simulink model "ale"  (R2022a)
settings: Solver=FixedStepAuto  StartTime=0.0  StopTime=10.0  FixedStep=framePeriod_s  RelTol=1e-3
undefined symbols (not defined in the file or in its folder): Aircraft, fire, framePeriod_s, led, throttle, turn
libraries: simulink x14, slpidlib x4, dspfdesign x1
(part 1 of 2)
settings Model: Creator=brian  LastModifiedBy=tuan
settings SolverCC: AlgebraicLoopSolver=TrustRegion
settings OptimizationCC: DefaultParameterBehavior=Inlined  GainParamInheritBuiltInType=on  UseFloatMulNetSlope=on  DefaultUnderspecifiedDataType=single  InlineInvariantSignals=on  PassReuseOutputArgsAs=Individual arguments  ZeroExternalMemoryAtStartup=off  ZeroInternalMemoryAtStartup=off  NoFixptDivByZeroProtection=on  EfficientFloat2IntCast=on  LifeSpan=1  OptimizeBlockOrder=speed  DifferentSizesBufferReuse=on  EfficientTunableParamExpr=on
settings DebuggingCC: ParameterTunabilityLossMsg=error  UnconnectedInputMsg=warning  UnconnectedOutputMsg=warning  UnconnectedLineMsg=warning  SFMachineParentedDataDiag=warning
settings HardwareCC: ProdBitPerPointer=32  ProdBitPerSizeT=32  ProdBitPerPtrDiffT=32  ProdLargestAtomicInteger=Long  ProdLargestAtomicFloat=Double  ProdWordSize=32  ProdLongLongMode=on  ProdHWDeviceType=NXP->Cortex-M4
settings ModelReferenceCC: ModelReferenceNumInstancesAllowed=Single
settings SFSimCC: SimParseCustomCode=off  MATLABDynamicMemAlloc=off
settings RTWCC: SystemTargetFile=ert.tlc  GenCodeOnly=on  TemplateMakefile=ert_default_tmf  RTWVerbose=off  BuildConfiguration=Faster Runs  TargetLang=C++  DLArmComputeVersion=19.05
settings CodeAppCC: ForceParamTrailComments=on  IgnoreCustomStorageClasses=off  OperatorAnnotations=on  SimulinkDataObjDesc=on  SFDataObjDesc=on  CustomSymbolStrGlobalVar=rt$N$M  CustomSymbolStrType=$N$M  CustomSymbolStrFcn=$N$M$F  CustomSymbolStrMacro=$N$M  InsertBlockDesc=on
settings ERTTargetCC: TargetLangStandard=C++03 (ISO)  IncludeMdlTerminateFcn=off  CombineSignalStateStructs=on  SuppressErrorStatus=on  SupportAbsoluteTime=off  CodeInterfacePackaging=C++ class  SupportNonFinite=off  SupportComplex=off  ERTHeaderFileRootName=autocode$E  ERTSourceFileRootName=autocode$E  InlinedParameterPlacement=NonHierarchical  RootIOFormat=Structure reference  ERTCustomFileTemplate=example_file_process.tlc  ERTFilePackagingFormat=Compact  ArrayContainerType=std::array

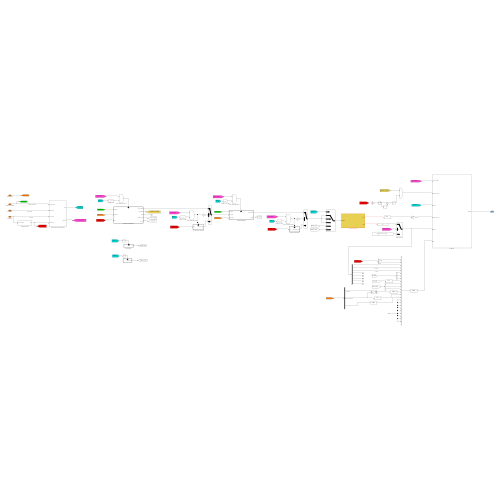
[thumbnail: Simulink's stored preview of the top-level diagram]
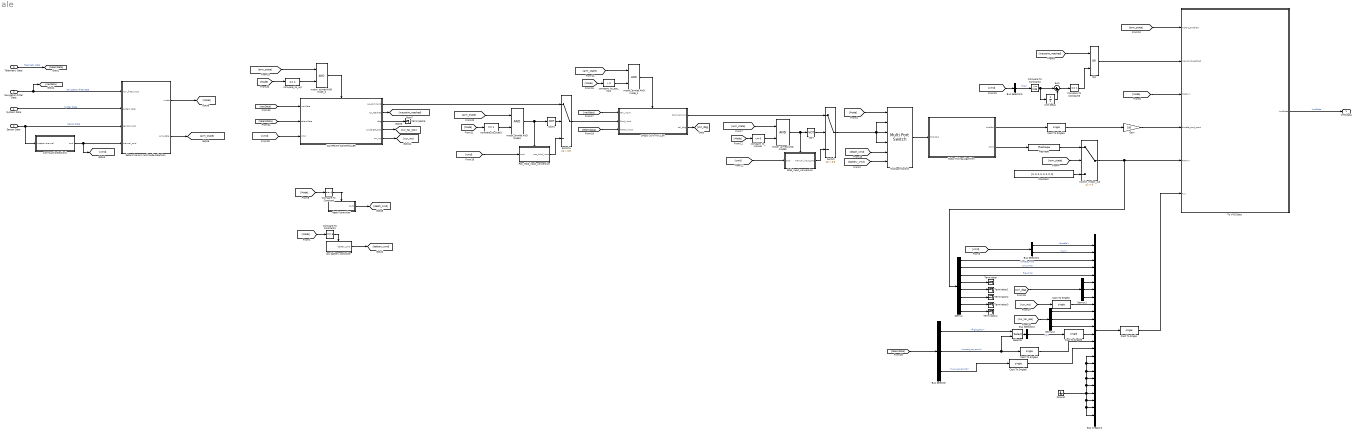
== system ale ==
  System Data : Inport  OutDataTypeStr=Bus: SysData  SampleTime=framePeriod_s  BusOutputAsStruct=on
  Sensor Data : Inport  Port=2  OutDataTypeStr=Bus: SensorData  SampleTime=framePeriod_s  BusOutputAsStruct=on
  Navigation Filter Data : Inport  Port=3  OutDataTypeStr=Bus: NavData  SampleTime=framePeriod_s  BusOutputAsStruct=on
  Telemetry Data : Inport  Port=4  OutDataTypeStr=Bus: TelemData  SampleTime=framePeriod_s  BusOutputAsStruct=on
  Bus Creator2 : BusCreator  Inputs=24
  Bus Selector : BusSelector  OutputSignals=flight_plan,current_waypoint,num_waypoints
  Bus Selector1 : BusSelector  OutputSignals=throttle,turn
  Bus Selector2 : BusSelector  OutputSignals=x
  Bus Selector3 : BusSelector  OutputSignals=fire
  Cast To Single{,1..5} (6 alike) : DataTypeConversion  OutDataTypeStr=single  SaturateOnIntegerOverflow=off  RndMeth=Floor
  Compare To Constant : simulink/Logic and Bit Operations/Compare To Constant  relop===  const=4  OutDataTypeStr=boolean
  Compare To Constant1 : simulink/Logic and Bit Operations/Compare To Constant  relop===  const=3  OutDataTypeStr=boolean
  Compare To Constant2 : simulink/Logic and Bit Operations/Compare To Constant  relop=>=  const=0.99  OutDataTypeStr=uint8
  Compare To Constant3 : simulink/Logic and Bit Operations/Compare To Constant  relop===  const=1  OutDataTypeStr=boolean
  Constant : Constant  Value=[0, 0, 0, 0, 0, 0, 0, 0]  OutDataTypeStr=single  SampleTime=framePeriod_s
  Demux : Demux  Outputs=8
  Demux1 : Demux  Outputs=3
  Demux2 : Demux  Outputs=3
  Gain : Gain  Gain=100
  Ground : Ground
  Motor Mixing Algorithm : Subsystem
  Multiport Switch : MultiPortSwitch  DataPortOrder=Specify indices  DataPortIndices={0, 1, 2, 3, 4}  DiagnosticForDefault=None  SaturateOnIntegerOverflow=off  InputSameDT=off
  NOT : Logic  Operator=NOT  IconShape=distinctive  AllPortsSameDT=off  OutDataTypeStr=boolean
  NOT1 : Logic  Operator=NOT  IconShape=distinctive  AllPortsSameDT=off  OutDataTypeStr=boolean
  OR : Logic  Operator=OR  IconShape=distinctive  AllPortsSameDT=off  OutDataTypeStr=boolean
  Pos_Hold_input_conversion : Subsystem
  Reshape : Reshape
  SPEED CONTROLLER : Subsystem
  Selector : Selector  IndexMode=Zero-based  InputPortWidth=100  IndexOptions=Index vector (port)  Indices=[1 3]  OutputSizes=1
  Stab_input_conversion : Subsystem
  Sum : Sum  Inputs=|+-
  Switch : Switch  Criteria=u2 > Threshold  Threshold=0.5  SaturateOnIntegerOverflow=off  InputSameDT=off
  Switch1 : Switch  Criteria=u2 > Threshold  Threshold=0.5  SaturateOnIntegerOverflow=off  InputSameDT=off
  Terminator{,1..5} (6 alike) : Terminator
  To VMS Data : Subsystem
  Unit Delay : UnitDelay  SampleTime=-1  HasFrameUpgradeWarning=on
  WAYPOINT CONTROLLER : Subsystem
  command selection1 : Subsystem
  compare_to_manual : simulink/Logic and Bit Operations/Compare To Constant  relop=<=  const=0  OutDataTypeStr=boolean
  compare_to_pos_hold : simulink/Logic and Bit Operations/Compare To Constant  relop=>  const=0  OutDataTypeStr=boolean
  compare_to_stab1 : simulink/Logic and Bit Operations/Compare To Constant  relop===  const=1  OutDataTypeStr=boolean
  compare_to_wp : simulink/Logic and Bit Operations/Compare To Constant  relop===  const=2  OutDataTypeStr=boolean
  death controller : Subsystem
  determine arm and mode selection : Subsystem
  low battery controller : Subsystem  TreatAsAtomicUnit=on
  motor_armed AND mode0 : Logic  IconShape=distinctive  AllPortsSameDT=off  OutDataTypeStr=boolean
  motor_armed AND mode1 : Logic  IconShape=distinctive  AllPortsSameDT=off  OutDataTypeStr=boolean
  motor_armed AND mode_1 : Logic  IconShape=distinctive  AllPortsSameDT=off  OutDataTypeStr=boolean
  motor_armed AND mode_2 : Logic  IconShape=distinctive  AllPortsSameDT=off  OutDataTypeStr=boolean
  switch_motor_out : Switch  Criteria=u2 > Threshold  SaturateOnIntegerOverflow=off  InputSameDT=off
  VMS Data : Outport  OutDataTypeStr=Bus: VmsData  SampleTime=framePeriod_s  BusOutputAsStruct=on
  wires:
  [Mode] -> To VMS Data/3(Mode in)
  Gain/1 -> To VMS Data/4(throttle_cmd_prcnt)
  Reshape/1 -> switch_motor_out/1
  Bus Selector1/1 -> Bus Creator2/1  "<throttle>"
  [arm_state] -> To VMS Data/1(motors_enabled)
  Ground/1 -> Bus Creator2/16, Bus Creator2/17, Bus Creator2/18, Bus Creator2/19, Bus Creator2/20, Bus Creator2/21, Bus Creator2/24, Bus Creator2/23, Bus Creator2/22
  [arm_state] -> switch_motor_out/2
  switch_motor_out/1 -> Demux/1, To VMS Data/5(PWM In)
  Constant/1 -> switch_motor_out/3
  Cast To Single/1 -> To VMS Data/6(Aux)
  Bus Creator2/1 -> Cast To Single/1
  Motor Mixing Algorithm/1(throttle) -> Cast To Single1/1
  Motor Mixing Algorithm/2(PWM) -> Reshape/1
  Cast To Single1/1 -> Gain/1
  To VMS Data/1(VmsData) -> VMS Data/1  "VmsData"
  Sensor Data/1 -> determine arm and mode selection/3(sensor_input), command selection1/1(inceptor channel)  "Sensor Data"
  Telemetry Data/1 -> [telemData]  "Telemetry Data"
  determine arm and mode selection/1(mode) -> [Mode]
  System Data/1 -> determine arm and mode selection/2(system data)  "Systen Data"
  determine arm and mode selection/2(arm_state) -> [arm_state]
  Navigation Filter Data/1 -> [navData], determine arm and mode selection/1(nav_filter_input)  "Navigation Filter Data"
  [cmd] -> Bus Selector1/1
  Bus Selector1/2 -> Bus Creator2/2  "<turn>"
  Demux/1 -> Bus Creator2/3  "throttle_mma"
  Demux/2 -> Bus Creator2/4  "turn_mma"
  Demux/3 -> Bus Creator2/5  "fire_mma"
  Demux/4 -> Terminator/1
  Demux/5 -> Terminator1/1
  Demux/6 -> Terminator2/1
  Demux/7 -> Terminator3/1
  Demux/8 -> Terminator4/1
  [Mode] -> Multiport Switch/1
  death controller/1(Out1) -> [death_cmd]
  [Mode] -> Compare To Constant/1
  Compare To Constant/1 -> death controller/Enable
  [Mode] -> Compare To Constant1/1
  Compare To Constant1/1 -> low battery controller/Enable
  low battery controller/1(battery_cmd) -> [battery_cmd]
  command selection1/1(cmd) -> determine arm and mode selection/4(manual_cmd), [cmd]
  Switch/1 -> Multiport Switch/2, Multiport Switch/4, Multiport Switch/3
  [Mode] -> compare_to_manual/1
  compare_to_manual/1 -> motor_armed AND mode0/2
  motor_armed AND mode0/1 -> Stab_input_conversion/Enable, NOT/1
  [arm_state] -> motor_armed AND mode0/1
  NOT/1 -> Switch/2
  [cmd] -> Stab_input_conversion/1(cmd)
  Stab_input_conversion/1(manual_input_cmd) -> Switch/3
  [navData] -> SPEED CONTROLLER/1(Nav_input)
  compare_to_pos_hold/1 -> motor_armed AND mode_1/2
  [arm_state] -> motor_armed AND mode_1/1
  [Mode] -> compare_to_pos_hold/1
  motor_armed AND mode_1/1 -> SPEED CONTROLLER/Enable
  SPEED CONTROLLER/1(Command out) -> Switch/1
  [Mode] -> compare_to_stab1/1
  motor_armed AND mode1/1 -> Pos_Hold_input_conversion/Enable, NOT1/1
  Switch1/1 -> SPEED CONTROLLER/2(Cmd_input)
  Pos_Hold_input_conversion/1(pos_hold_input) -> Switch1/3
  compare_to_stab1/1 -> motor_armed AND mode1/2
  NOT1/1 -> Switch1/2
  [cmd] -> Pos_Hold_input_conversion/1(cmd)
  [arm_state] -> motor_armed AND mode1/1
  [telemData] -> SPEED CONTROLLER/3(Telem_input)
  Multiport Switch/1 -> Motor Mixing Algorithm/1(MMA Bus)
  WAYPOINT CONTROLLER/1(wp_command) -> Switch1/1
  WAYPOINT CONTROLLER/2(wp_reached) -> [waypoint_reached]
  WAYPOINT CONTROLLER/3(dbg) -> Terminator5/1
  [arm_state] -> motor_armed AND mode_2/1
  compare_to_wp/1 -> motor_armed AND mode_2/2
  [Mode] -> compare_to_wp/1
  motor_armed AND mode_2/1 -> WAYPOINT CONTROLLER/Enable
  [telemData] -> WAYPOINT CONTROLLER/2(telemData)
  [navData] -> WAYPOINT CONTROLLER/1(navData)
  [cmd] -> WAYPOINT CONTROLLER/3(cmd)
  [battery_cmd] -> Multiport Switch/6
  [death_cmd] -> Multiport Switch/5
  SPEED CONTROLLER/2(ctrl_dbg) -> [ctrl_dbg]
  [ctrl_dbg] -> Demux1/1
  Demux1/1 -> Bus Creator2/6
  Demux1/2 -> Bus Creator2/7
  Demux1/3 -> Bus Creator2/8
  WAYPOINT CONTROLLER/4(cur_target_pos) -> [cur_tar_pos]
  WAYPOINT CONTROLLER/5(cur_wp) -> [cur_wp]
  [cur_wp] -> Cast To Single2/1
  Demux2/3 -> Bus Creator2/12
  Demux2/2 -> Bus Creator2/11
  Demux2/1 -> Bus Creator2/10
  [cur_tar_pos] -> Demux2/1
  Cast To Single2/1 -> Bus Creator2/9
  [telemData] -> Bus Selector/1
  Bus Selector/1 -> Selector/1  "<flight_plan>"
  Selector/1 -> Bus Selector2/1
  Bus Selector2/1 -> Cast To Single3/1  "<x>"
  Cast To Single3/1 -> Bus Creator2/13
  Bus Selector/2 -> Selector/2, Cast To Single4/1  "<current_waypoint>"
  [waypoint_reached] -> OR/1
  OR/1 -> To VMS Data/2(waypoint_reached)
  [cmd] -> Bus Selector3/1
  Bus Selector3/1 -> Compare To Constant2/1  "<fire>"
  Bus Selector/3 -> Cast To Single5/1  "<num_waypoints>"
  Cast To Single4/1 -> Bus Creator2/14
  Cast To Single5/1 -> Bus Creator2/15
  Compare To Constant2/1 -> Sum/1, Unit Delay/1
  Compare To Constant3/1 -> OR/2
  Sum/1 -> Compare To Constant3/1
  Unit Delay/1 -> Sum/2

== system ale/Motor Mixing Algorithm ==
  note: Other outputs are for fun things like Laser, Death or alive signal and speeker
  note: Motor output command is from -1 to 1
  note: this block map the control input to the correct hardware output signal. ie speed and turn command to the corresponding wheel speeds
  MMA Bus : Inport
  Bus Selector : BusSelector  OutputSignals=throttle,turn,fire,led
  Motor Mix : Constant  Value=Aircraft.Motor.mix  OutDataTypeStr=single  SampleTime=framePeriod_s
  Multiply : Product  Inputs=**  Multiplication=Matrix(*)  OutDataTypeStr=single
  Mux : Mux
  Reshape : Reshape  OutputDimensionality=Column vector (2-D)
  Saturation : Saturate  UpperLimit=1  LowerLimit=-1
  throttle : Outport
  PWM : Outport  Port=2
  wires:
  Mux/1 -> Reshape/1
  MMA Bus/1 -> Bus Selector/1
  Bus Selector/1 -> throttle/1, Mux/1  "<throttle>"
  Bus Selector/2 -> Mux/2  "<turn>"
  Multiply/1 -> Saturation/1  "Command"
  Reshape/1 -> Multiply/2
  Motor Mix/1 -> Multiply/1
  Bus Selector/3 -> Mux/3  "<fire>"
  Saturation/1 -> PWM/1
  Bus Selector/4 -> Mux/4  "<led>"

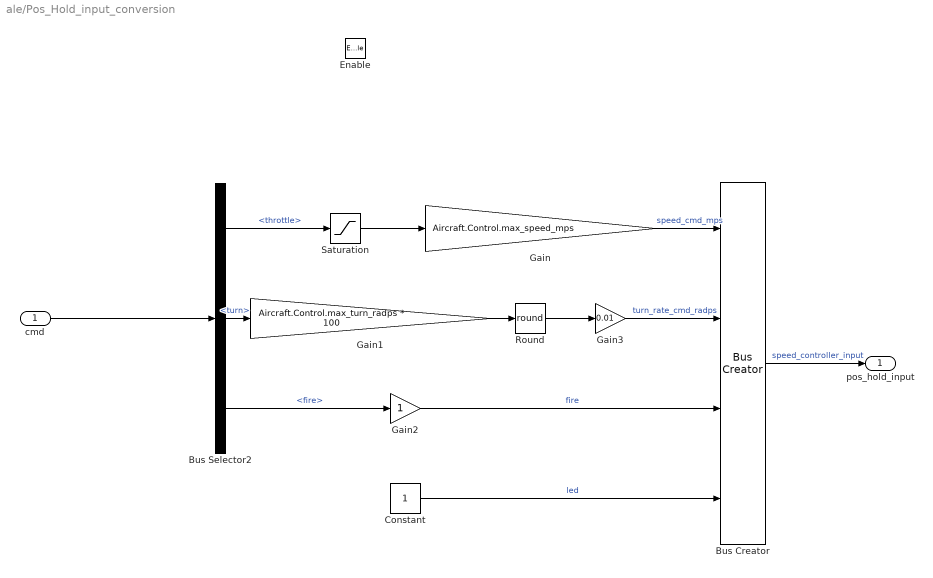
== system ale/Pos_Hold_input_conversion ==
  cmd : Inport
  Enable : EnablePort
  Bus Creator : BusCreator  Inputs=4
  Bus Selector2 : BusSelector  OutputSignals=throttle,turn,fire
  Constant : Constant  OutDataTypeStr=single
  Gain : Gain  Gain=Aircraft.Control.max_speed_mps
  Gain1 : Gain  Gain=Aircraft.Control.max_turn_radps * 100
  Gain2 : Gain
  Gain3 : Gain  Gain=0.01
  Round : Rounding  Operator=round
  Saturation : Saturate  UpperLimit=1  LowerLimit=0
  pos_hold_input : Outport
  wires:
  Bus Selector2/2 -> Gain1/1  "<turn>"
  Bus Creator/1 -> pos_hold_input/1  "speed_controller_input"
  Gain2/1 -> Bus Creator/3  "fire"
  Gain/1 -> Bus Creator/1  "speed_cmd_mps"
  Bus Selector2/3 -> Gain2/1  "<fire>"
  Constant/1 -> Bus Creator/4  "led"
  Bus Selector2/1 -> Saturation/1  "<throttle>"
  cmd/1 -> Bus Selector2/1
  Gain1/1 -> Round/1
  Round/1 -> Gain3/1
  Gain3/1 -> Bus Creator/2  "turn_rate_cmd_radps"
  Saturation/1 -> Gain/1

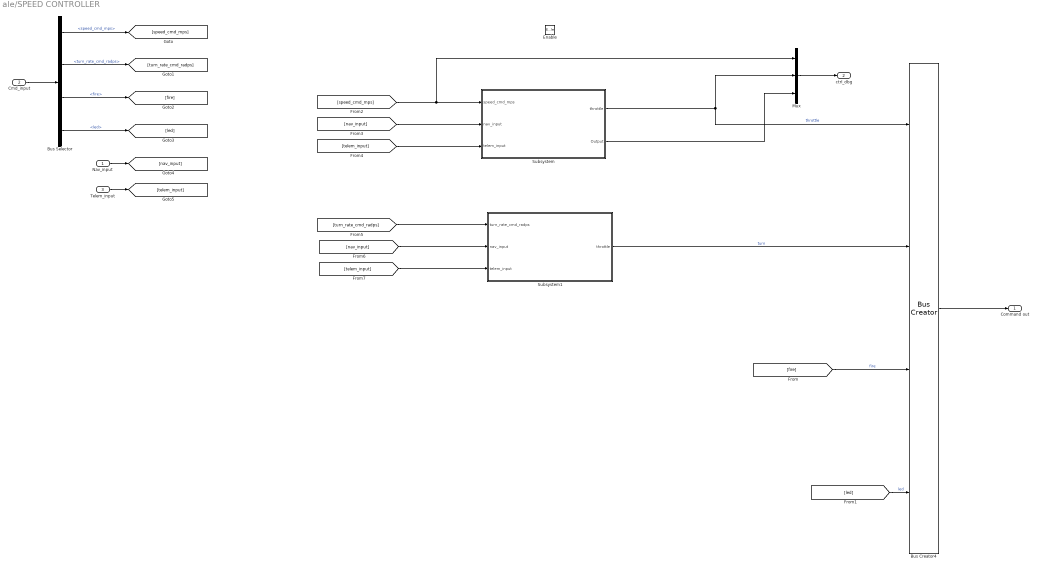
== system ale/SPEED CONTROLLER ==
  Nav_input : Inport
  Cmd_input : Inport  Port=2
  Telem_input : Inport  Port=3
  Enable : EnablePort  PropagateVarSize=During execution
  Bus Creator4 : BusCreator  Inputs=throttle,turn,fire,led
  Bus Selector : BusSelector  OutputSignals=speed_cmd_mps,turn_rate_cmd_radps,fire,led
  Mux : Mux  Inputs=3
  Subsystem : Subsystem
  Subsystem1 : Subsystem
  Command out : Outport
  ctrl_dbg : Outport  Port=2
  wires:
  Bus Creator4/1 -> Command out/1
  Cmd_input/1 -> Bus Selector/1
  [led] -> Bus Creator4/4  "led"
  Subsystem1/1(throttle) -> Bus Creator4/2  "turn"
  [fire] -> Bus Creator4/3  "fire"
  Bus Selector/1 -> [speed_cmd_mps]  "<speed_cmd_mps>"
  Bus Selector/4 -> [led]  "<led>"
  Bus Selector/3 -> [fire]  "<fire>"
  Bus Selector/2 -> [turn_rate_cmd_radps]  "<turn_rate_cmd_radps>"
  [speed_cmd_mps] -> Mux/1, Subsystem/1(speed_cmd_mps)
  Subsystem/1(throttle) -> Bus Creator4/1, Mux/2  "throttle"
  Nav_input/1 -> [nav_input]
  Telem_input/1 -> [telem_input]
  [nav_input] -> Subsystem/2(nav_input)
  [telem_input] -> Subsystem/3(telem_input)
  [turn_rate_cmd_radps] -> Subsystem1/1(turn_rate_cmd_radps)
  [nav_input] -> Subsystem1/2(nav_input)
  [telem_input] -> Subsystem1/3(telem_input)
  Mux/1 -> ctrl_dbg/1
  Subsystem/2(Output) -> Mux/3

== system ale/Stab_input_conversion ==
  cmd : Inport
  Enable : EnablePort
  Bus Creator : BusCreator  Inputs=4
  Bus Selector2 : BusSelector  OutputSignals=throttle,turn,fire
  Constant : Constant  OutDataTypeStr=single  SampleTime=framePeriod_s
  Gain : Gain
  Gain1 : Gain
  Gain2 : Gain
  manual_input_cmd : Outport
  wires:
  Bus Selector2/2 -> Gain1/1  "<turn>"
  Bus Creator/1 -> manual_input_cmd/1  "manual_input"
  Gain1/1 -> Bus Creator/2  "turn"
  cmd/1 -> Bus Selector2/1
  Bus Selector2/1 -> Gain/1  "<throttle>"
  Gain/1 -> Bus Creator/1  "throttle"
  Gain2/1 -> Bus Creator/3  "fire"
  Bus Selector2/3 -> Gain2/1  "<fire>"
  Constant/1 -> Bus Creator/4  "led"

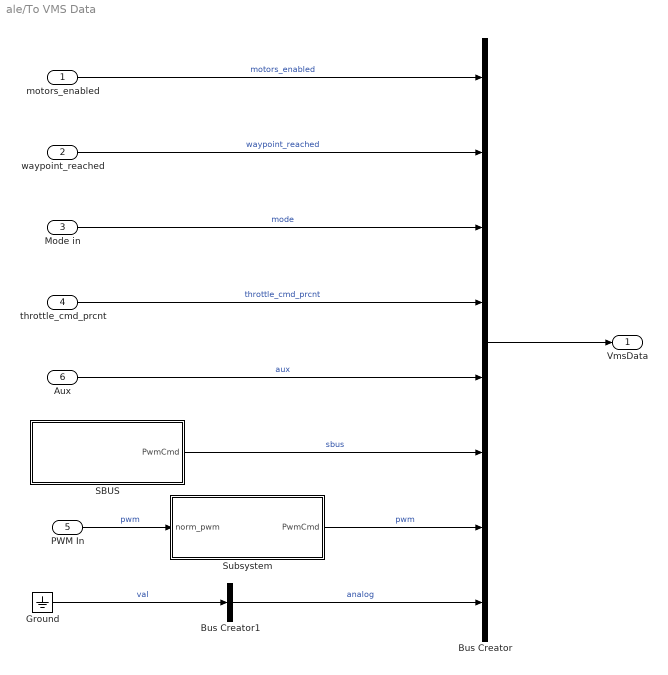
== system ale/To VMS Data ==
  motors_enabled : Inport
  waypoint_reached : Inport  Port=2
  Mode in : Inport  Port=3
  throttle_cmd_prcnt : Inport  Port=4
  PWM In : Inport  Port=5
  Aux : Inport  Port=6
  Bus Creator : BusCreator  Inputs=8  OutDataTypeStr=Bus: VmsData  NonVirtualBus=on
  Bus Creator1 : BusCreator  Inputs=1  OutDataTypeStr=Bus: AnalogData
  Ground : Ground
  "SBUS " : Subsystem
  Subsystem : Subsystem
  VmsData : Outport
  wires:
  waypoint_reached/1 -> Bus Creator/2  "waypoint_reached"
  Mode in/1 -> Bus Creator/3  "mode"
  motors_enabled/1 -> Bus Creator/1  "motors_enabled"
  Bus Creator/1 -> VmsData/1
  throttle_cmd_prcnt/1 -> Bus Creator/4  "throttle_cmd_prcnt"
  PWM In/1 -> Subsystem/1(norm_pwm)  "pwm"
  Subsystem/1(PwmCmd) -> Bus Creator/7  "pwm"
  Bus Creator1/1 -> Bus Creator/8  "analog"
  Ground/1 -> Bus Creator1/1  "val"
  Aux/1 -> Bus Creator/5  "aux"
  "SBUS "/1(PwmCmd) -> Bus Creator/6  "sbus"

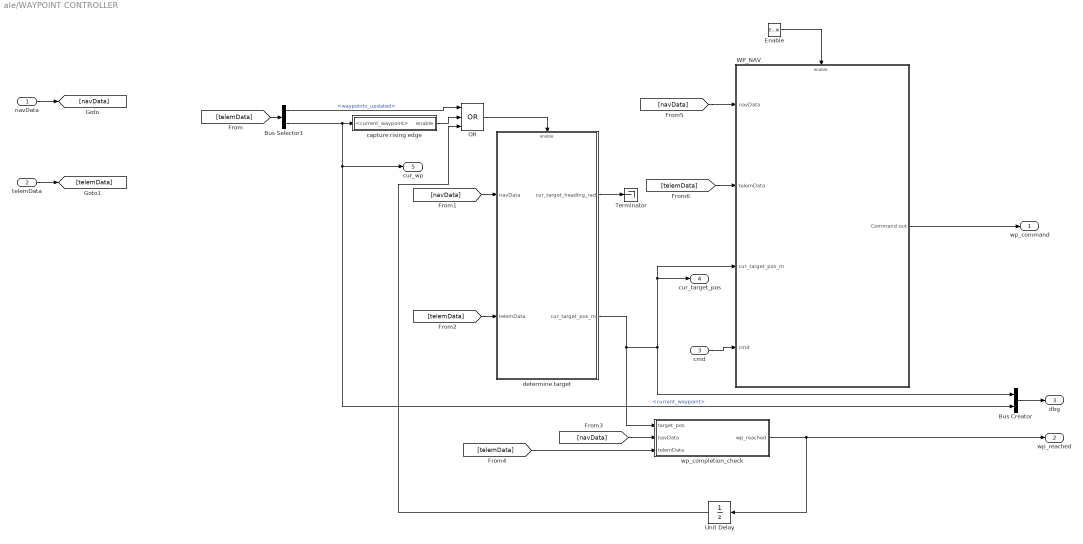
== system ale/WAYPOINT CONTROLLER ==
  navData : Inport
  telemData : Inport  Port=2
  cmd : Inport  Port=3
  Enable : EnablePort  ShowOutputPort=on
  Bus Creator : BusCreator  Inputs=2
  Bus Selector1 : BusSelector  OutputSignals=waypoints_updated,current_waypoint
  OR : Logic  Operator=OR  Inputs=3  IconShape=distinctive  AllPortsSameDT=off  OutDataTypeStr=boolean
  Terminator : Terminator
  Unit Delay : UnitDelay  SampleTime=-1  HasFrameUpgradeWarning=on
  WP_NAV : Subsystem
  capture rising edge : Subsystem
  determine target : Subsystem
  wp_completion_check : Subsystem
  wp_command : Outport
  wp_reached : Outport  Port=2
  dbg : Outport  Port=3
  cur_target_pos : Outport  Port=4
  cur_wp : Outport  Port=5
  wires:
  Enable/1 -> WP_NAV/Enable
  wp_completion_check/1(wp_reached) -> Unit Delay/1, wp_reached/1
  WP_NAV/1(Command out) -> wp_command/1
  determine target/2(cur_target_pos_m) -> wp_completion_check/1(target_pos), Bus Creator/1, WP_NAV/3(cur_target_pos_m), cur_target_pos/1
  Bus Selector1/2 -> cur_wp/1, Bus Creator/2, capture rising edge/1(<current_waypoint>)  "<current_waypoint>"
  Bus Creator/1 -> dbg/1
  OR/1 -> determine target/Enable
  Bus Selector1/1 -> OR/1  "<waypoints_updated>"
  capture rising edge/1(enable) -> OR/2
  navData/1 -> [navData]
  telemData/1 -> [telemData]
  [telemData] -> Bus Selector1/1
  [navData] -> determine target/1(navData)
  [telemData] -> determine target/2(telemData)
  [navData] -> wp_completion_check/2(navData)
  [telemData] -> wp_completion_check/3(telemData)
  [navData] -> WP_NAV/1(navData)
  determine target/1(cur_target_heading_rad) -> Terminator/1
  cmd/1 -> WP_NAV/4(cmd)
  [telemData] -> WP_NAV/2(telemData)
  Unit Delay/1 -> OR/3

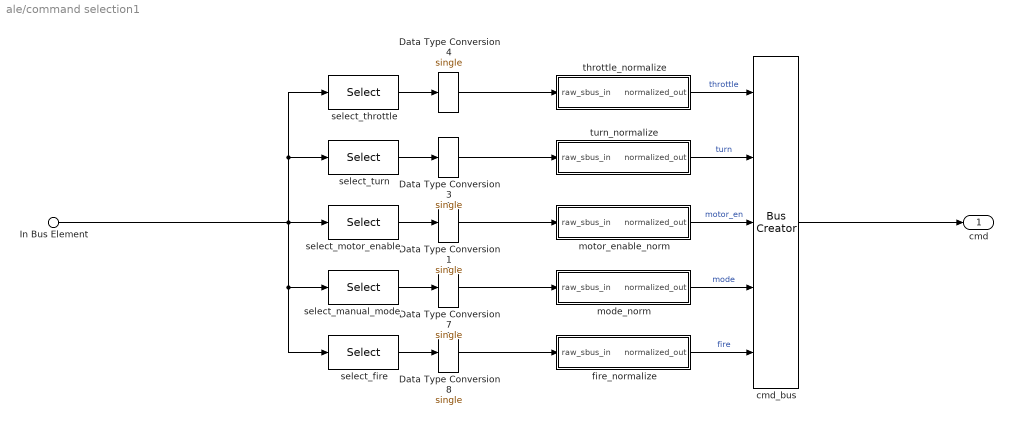
== system ale/command selection1 ==
  In Bus Element : Inport  PortName=inceptor channel  Element=inceptor.ch
  Data Type Conversion{1,3..4,7..8} (5 alike) : DataTypeConversion  OutDataTypeStr=single  SaturateOnIntegerOverflow=off  RndMeth=Floor
  cmd_bus : BusCreator  Inputs=5
  fire_normalize : Subsystem
  mode_norm : Subsystem
  motor_enable_norm : Subsystem
  select_fire : Selector  IndexOptions=Index vector (dialog)  Indices=Aircraft.Inceptor.fire  OutputSizes=1
  select_manual_mode : Selector  IndexOptions=Index vector (dialog)  Indices=Aircraft.Inceptor.mode0  OutputSizes=1
  select_motor_enable : Selector  IndexOptions=Index vector (dialog)  Indices=Aircraft.Inceptor.throttle_en  OutputSizes=1
  select_throttle : Selector  IndexOptions=Index vector (dialog)  Indices=Aircraft.Inceptor.throttle  OutputSizes=1
  select_turn : Selector  IndexOptions=Index vector (dialog)  Indices=Aircraft.Inceptor.turn  OutputSizes=1
  throttle_normalize : Subsystem
  turn_normalize : Subsystem
  cmd : Outport
  wires:
  select_throttle/1 -> Data Type Conversion4/1
  cmd_bus/1 -> cmd/1
  select_turn/1 -> Data Type Conversion3/1
  In Bus Element/1 -> select_fire/1, select_manual_mode/1, select_throttle/1, select_turn/1, select_motor_enable/1
  Data Type Conversion1/1 -> motor_enable_norm/1(raw_sbus_in)
  select_motor_enable/1 -> Data Type Conversion1/1
  Data Type Conversion7/1 -> mode_norm/1(raw_sbus_in)
  select_manual_mode/1 -> Data Type Conversion7/1
  select_fire/1 -> Data Type Conversion8/1
  Data Type Conversion8/1 -> fire_normalize/1(raw_sbus_in)
  Data Type Conversion4/1 -> throttle_normalize/1(raw_sbus_in)
  Data Type Conversion3/1 -> turn_normalize/1(raw_sbus_in)
  throttle_normalize/1(normalized_out) -> cmd_bus/1  "throttle"
  turn_normalize/1(normalized_out) -> cmd_bus/2  "turn"
  motor_enable_norm/1(normalized_out) -> cmd_bus/3  "motor_en"
  mode_norm/1(normalized_out) -> cmd_bus/4  "mode"
  fire_normalize/1(normalized_out) -> cmd_bus/5  "fire"

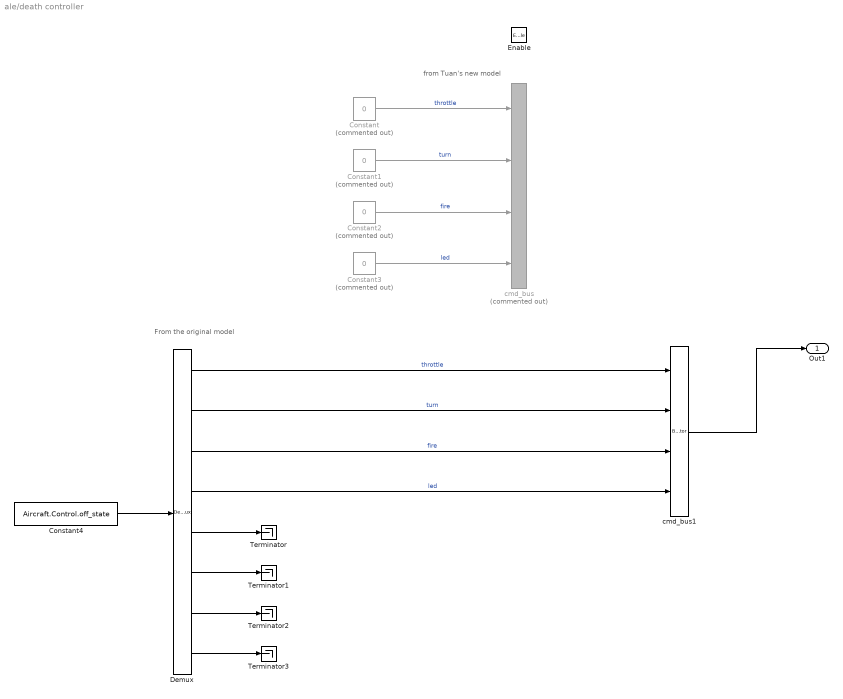
== system ale/death controller ==
  note: From the original model
  note: from Tuan's new model
  Enable : EnablePort
  Constant{,1..3} (4 alike) : Constant  Commented=on  Value=0  OutDataTypeStr=single  SampleTime=framePeriod_s
  Constant4 : Constant  Value=Aircraft.Control.off_state  OutDataTypeStr=single  SampleTime=framePeriod_s
  Demux : Demux  Outputs=8
  Terminator{,1..3} (4 alike) : Terminator
  cmd_bus : BusCreator  Commented=on  Inputs=4
  cmd_bus1 : BusCreator  Inputs=4
  Out1 : Outport
  wires:
  Constant/1 -> cmd_bus/1  "throttle"
  Constant1/1 -> cmd_bus/2  "turn"
  Constant2/1 -> cmd_bus/3  "fire"
  Constant3/1 -> cmd_bus/4  "led"
  Demux/2 -> cmd_bus1/2  "turn"
  Demux/7 -> Terminator2/1
  Demux/3 -> cmd_bus1/3  "fire"
  Demux/8 -> Terminator3/1
  Demux/1 -> cmd_bus1/1  "throttle"
  cmd_bus1/1 -> Out1/1
  Demux/4 -> cmd_bus1/4  "led"
  Demux/6 -> Terminator1/1
  Constant4/1 -> Demux/1
  Demux/5 -> Terminator/1

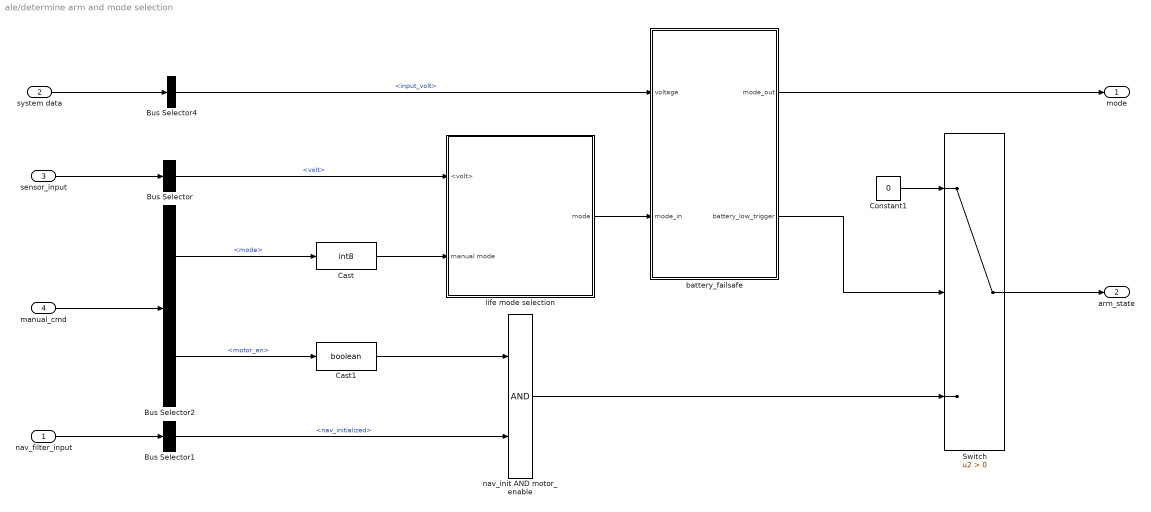
== system ale/determine arm and mode selection ==
  nav_filter_input : Inport
  system data : Inport  Port=2
  sensor_input : Inport  Port=3
  manual_cmd : Inport  Port=4
  Bus Selector : BusSelector  OutputSignals=adc.volt
  Bus Selector1 : BusSelector  OutputSignals=nav_initialized
  Bus Selector2 : BusSelector  OutputSignals=mode,motor_en
  Bus Selector4 : BusSelector  OutputSignals=input_volt
  Cast : DataTypeConversion  OutDataTypeStr=int8  RndMeth=Nearest  SaturateOnIntegerOverflow=off
  Cast1 : DataTypeConversion  OutDataTypeStr=boolean  SaturateOnIntegerOverflow=off  RndMeth=Floor
  Constant1 : Constant  Value=0  OutDataTypeStr=boolean  SampleTime=framePeriod_s
  Switch : Switch  Criteria=u2 > Threshold  SaturateOnIntegerOverflow=off  InputSameDT=off
  battery_failsafe : Subsystem
  life mode selection : Subsystem
  nav_init AND motor_enable : Logic  IconShape=distinctive  AllPortsSameDT=off  OutDataTypeStr=boolean
  mode : Outport
  arm_state : Outport  Port=2
  wires:
  Cast1/1 -> nav_init AND motor_enable/1
  nav_init AND motor_enable/1 -> Switch/3
  sensor_input/1 -> Bus Selector/1
  nav_filter_input/1 -> Bus Selector1/1
  Bus Selector1/1 -> nav_init AND motor_enable/2  "<nav_initialized>"
  Bus Selector/1 -> life mode selection/1(<volt>)  "<volt>"
  Cast/1 -> life mode selection/2(manual mode)
  life mode selection/1(mode) -> battery_failsafe/2(mode_in)
  battery_failsafe/1(mode_out) -> mode/1
  system data/1 -> Bus Selector4/1
  Bus Selector4/1 -> battery_failsafe/1(voltage)  "<input_volt>"
  Switch/1 -> arm_state/1
  battery_failsafe/2(battery_low_trigger) -> Switch/2
  Constant1/1 -> Switch/1
  manual_cmd/1 -> Bus Selector2/1
  Bus Selector2/1 -> Cast/1  "<mode>"
  Bus Selector2/2 -> Cast1/1  "<motor_en>"

== system ale/low battery controller ==
  Enable : EnablePort
  Cast : DataTypeConversion  OutDataTypeStr=single  SaturateOnIntegerOverflow=off  RndMeth=Floor
  Constant1 : Constant  OutDataTypeStr=single  SampleTime=framePeriod_s
  Constant4 : Constant  Value=0  OutDataTypeStr=single  SampleTime=framePeriod_s
  Constant5 : Constant  Value=0  OutDataTypeStr=single  SampleTime=framePeriod_s
  Discrete Pulse Generator : DiscretePulseGenerator  PulseType=Time based  PulseWidth=5
  cmd_bus : BusCreator  Inputs=4
  battery_cmd : Outport
  wires:
  cmd_bus/1 -> battery_cmd/1
  Discrete Pulse Generator/1 -> Cast/1  "fire"
  Constant4/1 -> cmd_bus/2  "turn"
  Constant5/1 -> cmd_bus/1  "throttle"
  Constant1/1 -> cmd_bus/4  "led"
  Cast/1 -> cmd_bus/3  "fire"

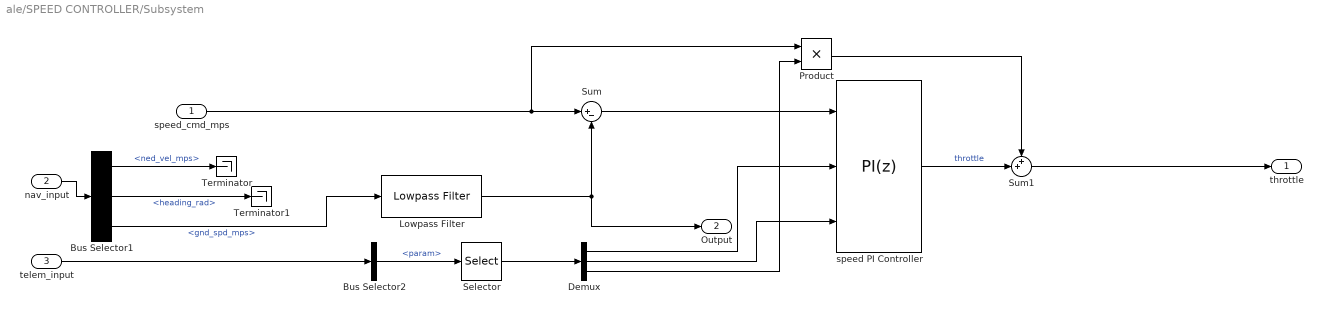
== system ale/SPEED CONTROLLER/Subsystem ==
  speed_cmd_mps : Inport
  nav_input : Inport  Port=2
  telem_input : Inport  Port=3
  Bus Selector1 : BusSelector  OutputSignals=ned_vel_mps,heading_rad,gnd_spd_mps
  Bus Selector2 : BusSelector  OutputSignals=param
  Demux : Demux  Outputs=3
  Lowpass Filter : dspfdesign/Lowpass Filter  FilterType=FIR  DesignForMinimumOrder=on  FilterOrder=50  PassbandFrequency=2  StopbandFrequency=5  PassbandRipple=0.1  StopbandAttenuation=10  InheritSampleRate=off  SampleRate=50  SimulateUsing=Code generation  roundingMode=Floor  coeffsDataTypeStr=fixdt(1,16)
  Product : Product
  Selector : Selector  IndexMode=Zero-based  IndexOptions=Index vector (dialog)  Indices=[0 1 2]  OutputSizes=1
  Sum : Sum  Inputs=|+-
  Sum1 : Sum  Inputs=++|
  Terminator : Terminator
  Terminator1 : Terminator
  speed PI Controller : slpidlib/PID Controller  Controller=PI  Form=Parallel  TimeDomain=Discrete-time  UseExternalTs=off  SampleTime=framePeriod_s  IntegratorMethod=Forward Euler  FilterMethod=Forward Euler  ControllerParametersSource=external  P=1  I=1  UseKiTs=off  D=0  N=100  UseFilter=on  TunerSelectOption=Transfer Function Based (PID Tuner App)  InitialConditionSource=internal  InitialConditionForIntegrator=0  InitialConditionForFilter=0  DifferentiatorICPrevScaledInput=0  ExternalReset=none  TrackingMode=off  Kt=1  LimitOutput=on  SatLimitsSource=internal  UpperSaturationLimit=1  LowerSaturationLimit=0  LinearizeAsGain=on  AntiWindupMode=clamping  Kb=1  POutMin=[]  POutMax=[]  IOutMin=[]  IOutMax=[]  DOutMin=[]  DOutMax=[]  NOutMin=[]  NOutMax=[]  SumOutMin=[]  SumOutMax=[]  SaturationOutMin=[]  SaturationOutMax=[]  PParamMin=[]  PParamMax=[]  IParamMin=[]  IParamMax=[]  DParamMin=[]  DParamMax=[]  NParamMin=[]  NParamMax=[]  KbParamMin=[]  KbParamMax=[]  KtParamMin=[]  KtParamMax=[]  KbOutMin=[]  KbOutMax=[]  KtOutMin=[]  KtOutMax=[]  IntegratorOutMin=[]  IntegratorOutMax=[]  FilterOutMin=[]  FilterOutMax=[]  SumI1OutMin=[]  SumI1OutMax=[]  SumI2OutMin=[]  SumI2OutMax=[]  SumI3OutMin=[]  SumI3OutMax=[]  SumI4OutMin=[]  SumI4OutMax=[]  SumDOutMin=[]  SumDOutMax=[]  DifferentiatorOutMin=[]  DifferentiatorOutMax=[]  FilterDiffOutCoefMin=[]  FilterDiffOutCoefMax=[]  ReciprocalOutMin=[]  ReciprocalOutMax=[]  SumDenOutMin=[]  SumDenOutMax=[]  SumNumOutMin=[]  SumNumOutMax=[]  DivideOutMin=[]  DivideOutMax=[]  UdiffTsProdOutMin=[]  UdiffTsProdOutMax=[]  NTsProdOutMin=[]  NTsProdOutMax=[]  UintegralTsProdOutMin=[]  UintegralTsProdOutMax=[]  UngainTsProdOutMin=[]  UngainTsProdOutMax=[]  IntegratorContinuousStateAttributes=''  IntegratorStateMustResolveToSignalObject=off  IntegratorRTWStateStorageClass=Auto  FilterContinuousStateAttributes=''  FilterStateMustResolveToSignalObject=off  FilterRTWStateStorageClass=Auto  ParallelPVariant=ExternalParameters  IdealPVariant=Disabled  IVariant=ExternalParameters  DVariant=Disabled  IntegratorVariant=Discrete  SatVariant=Enabled  AWVariant=DiscClampingParallel  PCopyVariant=Disabled  TRVariant=Disabled  FdbkBlocksVariant=Forward  IdealPFdbkVariant=Disabled  SatFdbkVariant=Disabled  DerivativeFilterVariant=Disabled  NVariant=Disabled  NCopyVariant=Disabled_SignalSpec  FilterICVariant=Disabled  IntegratorICVariant=InternalICs  ExternalResetVariant=Disabled  TRSumVariant=Passthrough  SumFdbkVariant=Disabled  SumVariant=Sum_PI  TsampFilterVariant=InternalTs  TsampNgainVariant=Passthrough  TsampIntegralVariant=Passthrough  ExternalSaturationOutDataTypeStr=Inherit: Same as second input  aMode=0
  throttle : Outport
  Output : Outport  Port=2
  wires:
  telem_input/1 -> Bus Selector2/1
  Sum/1 -> speed PI Controller/1
  nav_input/1 -> Bus Selector1/1
  Bus Selector2/1 -> Selector/1  "<param>"
  Demux/1 -> speed PI Controller/2
  Demux/2 -> speed PI Controller/3
  Selector/1 -> Demux/1
  Bus Selector1/1 -> Terminator/1  "<ned_vel_mps>"
  Bus Selector1/2 -> Terminator1/1  "<heading_rad>"
  speed_cmd_mps/1 -> Product/1, Sum/1
  Lowpass Filter/1 -> Output/1, Sum/2
  Bus Selector1/3 -> Lowpass Filter/1  "<gnd_spd_mps>"
  speed PI Controller/1 -> Sum1/2  "throttle"
  Sum1/1 -> throttle/1
  Demux/3 -> Product/2
  Product/1 -> Sum1/1

== system ale/SPEED CONTROLLER/Subsystem1 ==
  turn_rate_cmd_radps : Inport
  nav_input : Inport  Port=2
  telem_input : Inport  Port=3
  Bus Selector1 : BusSelector  OutputSignals=gyro_radps
  Bus Selector2 : BusSelector  OutputSignals=param
  Demux : Demux  Outputs=2
  Selector : Selector  IndexMode=Zero-based  InputPortWidth=24  IndexOptions=Index vector (dialog)  Indices=[3 4]  OutputSizes=1
  Selector1 : Selector  InputPortWidth=3  IndexOptions=Index vector (dialog)  Indices=3  OutputSizes=1
  Sum : Sum  Inputs=|+-
  turn_rate PI Controller : slpidlib/PID Controller  Controller=PI  Form=Parallel  TimeDomain=Discrete-time  UseExternalTs=off  SampleTime=framePeriod_s  IntegratorMethod=Forward Euler  FilterMethod=Forward Euler  ControllerParametersSource=external  P=1  I=1  UseKiTs=off  D=0  N=100  UseFilter=on  TunerSelectOption=Transfer Function Based (PID Tuner App)  InitialConditionSource=internal  InitialConditionForIntegrator=0  InitialConditionForFilter=0  DifferentiatorICPrevScaledInput=0  ExternalReset=none  TrackingMode=off  Kt=1  LimitOutput=on  SatLimitsSource=internal  UpperSaturationLimit=1  LowerSaturationLimit=-1  LinearizeAsGain=on  AntiWindupMode=clamping  Kb=1  POutMin=[]  POutMax=[]  IOutMin=[]  IOutMax=[]  DOutMin=[]  DOutMax=[]  NOutMin=[]  NOutMax=[]  SumOutMin=[]  SumOutMax=[]  SaturationOutMin=[]  SaturationOutMax=[]  PParamMin=[]  PParamMax=[]  IParamMin=[]  IParamMax=[]  DParamMin=[]  DParamMax=[]  NParamMin=[]  NParamMax=[]  KbParamMin=[]  KbParamMax=[]  KtParamMin=[]  KtParamMax=[]  KbOutMin=[]  KbOutMax=[]  KtOutMin=[]  KtOutMax=[]  IntegratorOutMin=[]  IntegratorOutMax=[]  FilterOutMin=[]  FilterOutMax=[]  SumI1OutMin=[]  SumI1OutMax=[]  SumI2OutMin=[]  SumI2OutMax=[]  SumI3OutMin=[]  SumI3OutMax=[]  SumI4OutMin=[]  SumI4OutMax=[]  SumDOutMin=[]  SumDOutMax=[]  DifferentiatorOutMin=[]  DifferentiatorOutMax=[]  FilterDiffOutCoefMin=[]  FilterDiffOutCoefMax=[]  ReciprocalOutMin=[]  ReciprocalOutMax=[]  SumDenOutMin=[]  SumDenOutMax=[]  SumNumOutMin=[]  SumNumOutMax=[]  DivideOutMin=[]  DivideOutMax=[]  UdiffTsProdOutMin=[]  UdiffTsProdOutMax=[]  NTsProdOutMin=[]  NTsProdOutMax=[]  UintegralTsProdOutMin=[]  UintegralTsProdOutMax=[]  UngainTsProdOutMin=[]  UngainTsProdOutMax=[]  IntegratorContinuousStateAttributes=''  IntegratorStateMustResolveToSignalObject=off  IntegratorRTWStateStorageClass=Auto  FilterContinuousStateAttributes=''  FilterStateMustResolveToSignalObject=off  FilterRTWStateStorageClass=Auto  ParallelPVariant=ExternalParameters  IdealPVariant=Disabled  IVariant=ExternalParameters  DVariant=Disabled  IntegratorVariant=Discrete  SatVariant=Enabled  AWVariant=DiscClampingParallel  PCopyVariant=Disabled  TRVariant=Disabled  FdbkBlocksVariant=Forward  IdealPFdbkVariant=Disabled  SatFdbkVariant=Disabled  DerivativeFilterVariant=Disabled  NVariant=Disabled  NCopyVariant=Disabled_SignalSpec  FilterICVariant=Disabled  IntegratorICVariant=InternalICs  ExternalResetVariant=Disabled  TRSumVariant=Passthrough  SumFdbkVariant=Disabled  SumVariant=Sum_PI  TsampFilterVariant=InternalTs  TsampNgainVariant=Passthrough  TsampIntegralVariant=Passthrough  ExternalSaturationOutDataTypeStr=Inherit: Same as second input  aMode=0
  throttle : Outport
  wires:
  turn_rate_cmd_radps/1 -> Sum/1
  telem_input/1 -> Bus Selector2/1
  Selector1/1 -> Sum/2
  Sum/1 -> turn_rate PI Controller/1
  nav_input/1 -> Bus Selector1/1
  Bus Selector2/1 -> Selector/1  "<param>"
  turn_rate PI Controller/1 -> throttle/1  "turn"
  Bus Selector1/1 -> Selector1/1  "<gyro_radps>"
  Selector/1 -> Demux/1
  Demux/1 -> turn_rate PI Controller/2
  Demux/2 -> turn_rate PI Controller/3

== system ale/To VMS Data/SBUS  ==
  Bus Creator : BusCreator  Inputs=4  OutDataTypeStr=Bus: SbusCmd
  Constant : Constant  OutDataTypeStr=boolean
  Constant1 : Constant  OutDataTypeStr=boolean
  Ground : Ground
  Ground1 : Ground
  PwmCmd : Outport
  wires:
  Bus Creator/1 -> PwmCmd/1
  Constant/1 -> Bus Creator/1  "ch17"
  Constant1/1 -> Bus Creator/2  "ch18"
  Ground/1 -> Bus Creator/3  "cnt"
  Ground1/1 -> Bus Creator/4  "cmd"

== system ale/To VMS Data/Subsystem ==
  note: cmd - output to feed to the simulator
  note: cnt - pwm output to actual hardware
  norm_pwm : Inport
  Bus Creator : BusCreator  Inputs=2  OutDataTypeStr=Bus: PwmCmd  NonVirtualBus=on
      settings: InheritFromInputs=off
  MATLAB Function : MATLAB Function  TreatAsAtomicUnit=on
  PwmCmd : Outport
  wires:
  Bus Creator/1 -> PwmCmd/1
  norm_pwm/1 -> Bus Creator/2, MATLAB Function/1(x)  "cmd"
  MATLAB Function/1(y_cnt) -> Bus Creator/1  "cnt"

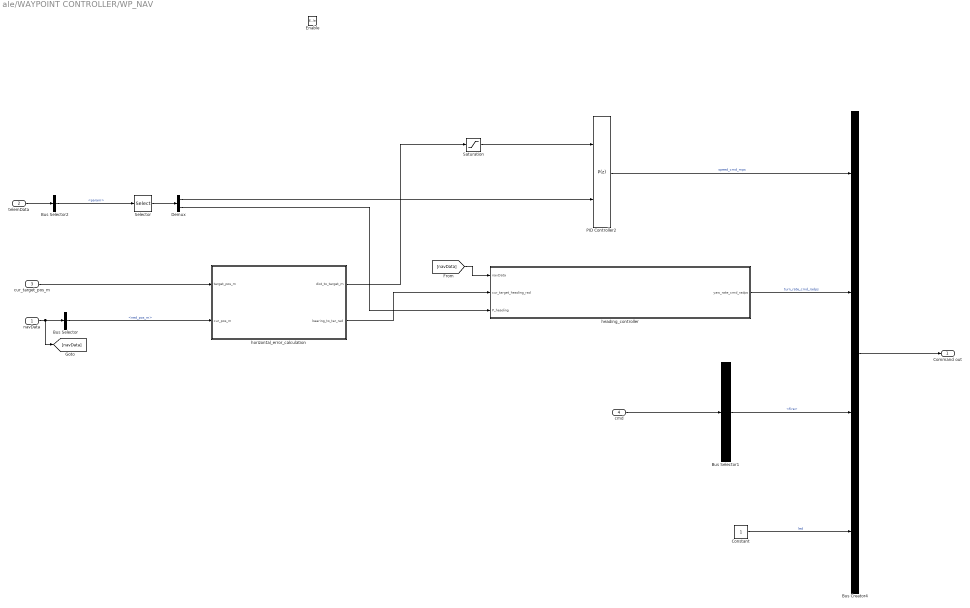
== system ale/WAYPOINT CONTROLLER/WP_NAV ==
  navData : Inport
  telemData : Inport  Port=2
  cur_target_pos_m : Inport  Port=3
  cmd : Inport  Port=4
  Enable : EnablePort
  Bus Creator4 : BusCreator  Inputs=4
  Bus Selector : BusSelector  OutputSignals=ned_pos_m
  Bus Selector1 : BusSelector  OutputSignals=fire
  Bus Selector2 : BusSelector  OutputSignals=param
  Constant : Constant  OutDataTypeStr=single
  Demux : Demux  Outputs=2
  PID Controller2 : slpidlib/PID Controller  Controller=P  Form=Parallel  TimeDomain=Discrete-time  UseExternalTs=off  SampleTime=framePeriod_s  IntegratorMethod=Forward Euler  FilterMethod=Forward Euler  ControllerParametersSource=external  P=0.335  I=0.005  UseKiTs=off  D=0  N=100  UseFilter=off  TunerSelectOption=Transfer Function Based (PID Tuner App)  InitialConditionSource=internal  InitialConditionForIntegrator=0  InitialConditionForFilter=0  DifferentiatorICPrevScaledInput=0  ExternalReset=none  TrackingMode=off  Kt=1  LimitOutput=on  SatLimitsSource=internal  UpperSaturationLimit=Aircraft.Control.max_speed_mps  LowerSaturationLimit=0  LinearizeAsGain=off  AntiWindupMode=clamping  Kb=1  POutMin=[]  POutMax=[]  IOutMin=[]  IOutMax=[]  DOutMin=[]  DOutMax=[]  NOutMin=[]  NOutMax=[]  SumOutMin=[]  SumOutMax=[]  SaturationOutMin=[]  SaturationOutMax=[]  PParamMin=[]  PParamMax=[]  IParamMin=[]  IParamMax=[]  DParamMin=[]  DParamMax=[]  NParamMin=[]  NParamMax=[]  KbParamMin=[]  KbParamMax=[]  KtParamMin=[]  KtParamMax=[]  KbOutMin=[]  KbOutMax=[]  KtOutMin=[]  KtOutMax=[]  IntegratorOutMin=[]  IntegratorOutMax=[]  FilterOutMin=[]  FilterOutMax=[]  SumI1OutMin=[]  SumI1OutMax=[]  SumI2OutMin=[]  SumI2OutMax=[]  SumI3OutMin=[]  SumI3OutMax=[]  SumI4OutMin=[]  SumI4OutMax=[]  SumDOutMin=[]  SumDOutMax=[]  DifferentiatorOutMin=[]  DifferentiatorOutMax=[]  FilterDiffOutCoefMin=[]  FilterDiffOutCoefMax=[]  ReciprocalOutMin=[]  ReciprocalOutMax=[]  SumDenOutMin=[]  SumDenOutMax=[]  SumNumOutMin=[]  SumNumOutMax=[]  DivideOutMin=[]  DivideOutMax=[]  UdiffTsProdOutMin=[]  UdiffTsProdOutMax=[]  NTsProdOutMin=[]  NTsProdOutMax=[]  UintegralTsProdOutMin=[]  UintegralTsProdOutMax=[]  UngainTsProdOutMin=[]  UngainTsProdOutMax=[]  IntegratorContinuousStateAttributes=''  IntegratorStateMustResolveToSignalObject=off  IntegratorRTWStateStorageClass=Auto  FilterContinuousStateAttributes=''  FilterStateMustResolveToSignalObject=off  FilterRTWStateStorageClass=Auto  ParallelPVariant=ExternalParameters  IdealPVariant=Disabled  IVariant=Disabled  DVariant=Disabled  IntegratorVariant=Disabled  SatVariant=Enabled  AWVariant=Disabled  PCopyVariant=Disabled  TRVariant=Disabled  FdbkBlocksVariant=Forward  IdealPFdbkVariant=Disabled  SatFdbkVariant=Disabled  DerivativeFilterVariant=Disabled  NVariant=Disabled  NCopyVariant=Disabled_SignalSpec  FilterICVariant=Disabled  IntegratorICVariant=Disabled  ExternalResetVariant=Disabled  TRSumVariant=Passthrough  SumFdbkVariant=Disabled  SumVariant=Passthrough_P  TsampFilterVariant=InternalTs  TsampNgainVariant=Passthrough  TsampIntegralVariant=Disabled_SignalSpec  ExternalSaturationOutDataTypeStr=Inherit: Same as second input  aMode=0
  Saturation : Saturate  UpperLimit=20  LowerLimit=0
  Selector : Selector  IndexMode=Zero-based  InputPortWidth=24  IndexOptions=Index vector (dialog)  Indices=[5 6]  OutputSizes=1
  heading_controller : Subsystem
  "horizontal_error_calculation " : Subsystem
  Command out : Outport
  wires:
  Bus Creator4/1 -> Command out/1
  cur_target_pos_m/1 -> "horizontal_error_calculation "/1(target_pos_m)
  navData/1 -> [navData], Bus Selector/1
  Bus Selector/1 -> "horizontal_error_calculation "/2(cur_pos_m)  "<ned_pos_m>"
  "horizontal_error_calculation "/2(bearing_to_tar_rad) -> heading_controller/2(cur_target_heading_rad)
  [navData] -> heading_controller/1(navData)
  Demux/1 -> PID Controller2/2
  "horizontal_error_calculation "/1(dist_to_target_m) -> Saturation/1
  Saturation/1 -> PID Controller2/1
  PID Controller2/1 -> Bus Creator4/1  "speed_cmd_mps"
  heading_controller/1(yaw_rate_cmd_radps) -> Bus Creator4/2  "turn_rate_cmd_radps"
  cmd/1 -> Bus Selector1/1
  Bus Selector1/1 -> Bus Creator4/3  "<fire>"
  Constant/1 -> Bus Creator4/4  "led"
  telemData/1 -> Bus Selector2/1
  Bus Selector2/1 -> Selector/1  "<param>"
  Selector/1 -> Demux/1
  Demux/2 -> heading_controller/3(P_heading)

== system ale/WAYPOINT CONTROLLER/capture rising edge ==
  <current_waypoint> : Inport
  Detect Change1 : simulink/Logic and Bit Operations/Detect Change  vinit=-1  OutDataTypeStr=boolean
  enable : Outport
  wires:
  <current_waypoint>/1 -> Detect Change1/1
  Detect Change1/1 -> enable/1

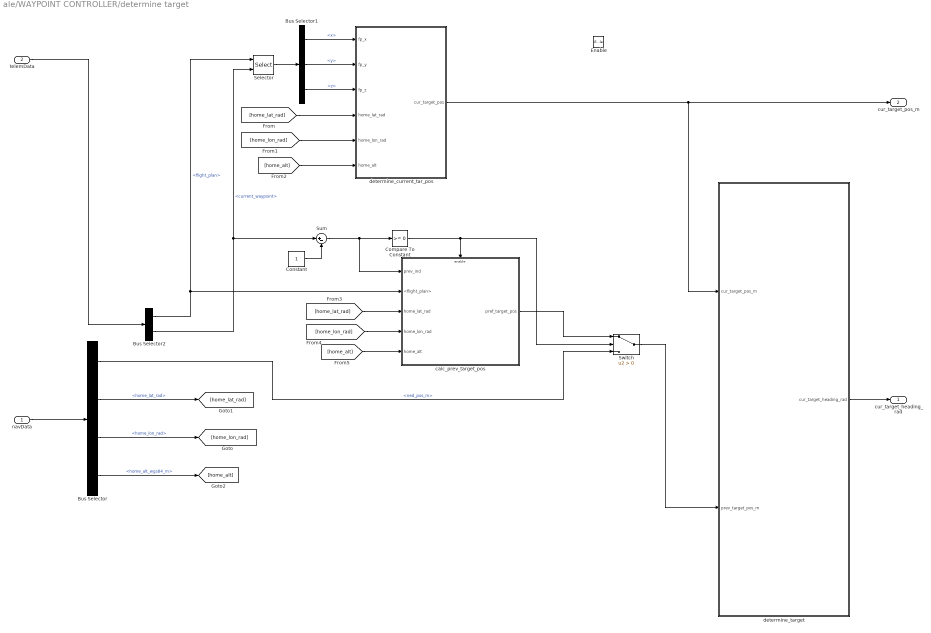
== system ale/WAYPOINT CONTROLLER/determine target ==
  navData : Inport
  telemData : Inport  Port=2
  Enable : EnablePort
  Bus Selector : BusSelector  OutputSignals=ned_pos_m,home_lat_rad,home_lon_rad,home_alt_wgs84_m
  Bus Selector1 : BusSelector  OutputSignals=x,y,z
  Bus Selector2 : BusSelector  OutputSignals=flight_plan,current_waypoint
  Compare To Constant : simulink/Logic and Bit Operations/Compare To Constant  relop=>=  const=0  OutDataTypeStr=boolean
  Constant : Constant
  Selector : Selector  IndexMode=Zero-based  InputPortWidth=100  IndexOptions=Index vector (port)  Indices=[1 3]  OutputSizes=1
  Sum : Sum  Inputs=|+-
  Switch : Switch  Criteria=u2 > Threshold  SaturateOnIntegerOverflow=off  InputSameDT=off
  calc_prev_target_pos : Subsystem
  determine_current_tar_pos : MATLAB Function  TreatAsAtomicUnit=on
  determine_target : MATLAB Function  TreatAsAtomicUnit=on
  cur_target_heading_rad : Outport
  cur_target_pos_m : Outport  Port=2
  wires:
  determine_current_tar_pos/1(cur_target_pos) -> cur_target_pos_m/1, determine_target/1(cur_target_pos_m)
  determine_target/1(cur_target_heading_rad) -> cur_target_heading_rad/1
  navData/1 -> Bus Selector/1
  Bus Selector2/2 -> Selector/2, Sum/1  "<current_waypoint>"
  Bus Selector/2 -> [home_lat_rad]  "<home_lat_rad>"
  Bus Selector2/1 -> Selector/1, calc_prev_target_pos/2(<flight_plan>)  "<flight_plan>"
  Bus Selector/3 -> [home_lon_rad]  "<home_lon_rad>"
  Bus Selector/4 -> [home_alt]  "<home_alt_wgs84_m>"
  Bus Selector/1 -> Switch/3  "<ned_pos_m>"
  Selector/1 -> Bus Selector1/1
  Bus Selector1/3 -> determine_current_tar_pos/3(fp_z)  "<z>"
  Bus Selector1/2 -> determine_current_tar_pos/2(fp_y)  "<y>"
  Bus Selector1/1 -> determine_current_tar_pos/1(fp_x)  "<x>"
  [home_lat_rad] -> determine_current_tar_pos/4(home_lat_rad)
  [home_lon_rad] -> determine_current_tar_pos/5(home_lon_rad)
  [home_alt] -> determine_current_tar_pos/6(home_alt)
  Constant/1 -> Sum/2
  Sum/1 -> calc_prev_target_pos/1(prev_ind), Compare To Constant/1
  [home_lat_rad] -> calc_prev_target_pos/3(home_lat_rad)
  [home_lon_rad] -> calc_prev_target_pos/4(home_lon_rad)
  [home_alt] -> calc_prev_target_pos/5(home_alt)
  Compare To Constant/1 -> Switch/2, calc_prev_target_pos/Enable
  calc_prev_target_pos/1(pref_target_pos) -> Switch/1
  Switch/1 -> determine_target/2(prev_target_pos_m)
  telemData/1 -> Bus Selector2/1

== system ale/WAYPOINT CONTROLLER/wp_completion_check ==
  note: Output wp_reached cmd only when distance between current pos and target pos is less than wp_radius.
  target_pos : Inport
  navData : Inport  Port=2
  telemData : Inport  Port=3
  Bus Selector : BusSelector  OutputSignals=ned_pos_m
  Bus Selector1 : BusSelector  OutputSignals=autocontinue
  Bus Selector2 : BusSelector  OutputSignals=flight_plan,current_waypoint,param
  Constant : Constant  Value=10
  Selector : Selector  IndexMode=Zero-based  InputPortWidth=100  IndexOptions=Index vector (port)  Indices=[1 3]  OutputSizes=1
  Selector1 : Selector  IndexMode=Zero-based  InputPortWidth=24  IndexOptions=Index vector (port)  Indices=10  OutputSizes=1
  check_wp_reached : MATLAB Function  TreatAsAtomicUnit=on
  wp_reached : Outport
  wires:
  Bus Selector/1 -> check_wp_reached/2(ned_pos)  "<ned_pos_m>"
  target_pos/1 -> check_wp_reached/1(target_pos)
  Bus Selector2/1 -> Selector/1  "<flight_plan>"
  Bus Selector2/2 -> Selector/2  "<current_waypoint>"
  Selector1/1 -> check_wp_reached/4(Aircraft_Control_wp_radius)  "wp_radius"
  check_wp_reached/1(reached) -> wp_reached/1
  Selector/1 -> Bus Selector1/1
  Bus Selector1/1 -> check_wp_reached/3(autocontinue)  "<autocontinue>"
  Bus Selector2/3 -> Selector1/1  "<param>"
  Constant/1 -> Selector1/2
  navData/1 -> Bus Selector/1
  telemData/1 -> Bus Selector2/1

== system ale/command selection1/fire_normalize ==
  raw_sbus_in : Inport
  Constant : Constant  Value=172  OutDataTypeStr=single
  Constant1 : Constant  Value=-1  OutDataTypeStr=single
  Constant2 : Constant  OutDataTypeStr=single
  Constant3 : Constant  Value=1811  OutDataTypeStr=single
  remap : MATLAB Function  TreatAsAtomicUnit=on
  normalized_out : Outport
  wires:
  raw_sbus_in/1 -> remap/1(raw_in)
  remap/1(norm_out) -> normalized_out/1
  Constant/1 -> remap/2(in_min)
  Constant3/1 -> remap/3(in_max)
  Constant1/1 -> remap/4(out_min)
  Constant2/1 -> remap/5(out_max)

== system ale/command selection1/mode_norm ==
  raw_sbus_in : Inport
  Constant : Constant  Value=172  OutDataTypeStr=single
  Constant1 : Constant  Value=0  OutDataTypeStr=single
  Constant2 : Constant  Value=2  OutDataTypeStr=single
  Constant3 : Constant  Value=1811  OutDataTypeStr=single
  remap : MATLAB Function  TreatAsAtomicUnit=on
  normalized_out : Outport
  wires:
  raw_sbus_in/1 -> remap/1(raw_in)
  remap/1(norm_out) -> normalized_out/1
  Constant/1 -> remap/2(in_min)
  Constant3/1 -> remap/3(in_max)
  Constant1/1 -> remap/4(out_min)
  Constant2/1 -> remap/5(out_max)

== system ale/command selection1/motor_enable_norm ==
  raw_sbus_in : Inport
  Constant : Constant  Value=172  OutDataTypeStr=single
  Constant1 : Constant  Value=0  OutDataTypeStr=single
  Constant2 : Constant  OutDataTypeStr=single
  Constant3 : Constant  Value=1811  OutDataTypeStr=single
  remap : MATLAB Function  TreatAsAtomicUnit=on
  normalized_out : Outport
  wires:
  Constant2/1 -> remap/5(out_max)
  Constant1/1 -> remap/4(out_min)
  Constant3/1 -> remap/3(in_max)
  Constant/1 -> remap/2(in_min)
  remap/1(norm_out) -> normalized_out/1
  raw_sbus_in/1 -> remap/1(raw_in)

== system ale/command selection1/throttle_normalize ==
  raw_sbus_in : Inport
  Constant : Constant  Value=172  OutDataTypeStr=single
  Constant1 : Constant  Value=-1  OutDataTypeStr=single
  Constant2 : Constant  OutDataTypeStr=single
  Constant3 : Constant  Value=1811  OutDataTypeStr=single
  remap : MATLAB Function  TreatAsAtomicUnit=on
  normalized_out : Outport
  wires:
  raw_sbus_in/1 -> remap/1(raw_in)
  remap/1(norm_out) -> normalized_out/1
  Constant/1 -> remap/2(in_min)
  Constant3/1 -> remap/3(in_max)
  Constant1/1 -> remap/4(out_min)
  Constant2/1 -> remap/5(out_max)

== system ale/command selection1/turn_normalize ==
  raw_sbus_in : Inport
  Constant : Constant  Value=172  OutDataTypeStr=single
  Constant1 : Constant  Value=-1  OutDataTypeStr=single
  Constant2 : Constant  OutDataTypeStr=single
  Constant3 : Constant  Value=1811  OutDataTypeStr=single
  remap : MATLAB Function  TreatAsAtomicUnit=on
  normalized_out : Outport
  wires:
  raw_sbus_in/1 -> remap/1(raw_in)
  remap/1(norm_out) -> normalized_out/1
  Constant/1 -> remap/2(in_min)
  Constant3/1 -> remap/3(in_max)
  Constant1/1 -> remap/4(out_min)
  Constant2/1 -> remap/5(out_max)

== system ale/determine arm and mode selection/battery_failsafe ==
  voltage : Inport
  mode_in : Inport  Port=2
  Compare To Constant3 : simulink/Logic and Bit Operations/Compare To Constant  relop=<=  const=3.2 * 3  OutDataTypeStr=boolean
  Constant : Constant  Value=3  OutDataTypeStr=int8  SampleTime=framePeriod_s
  Switch : Switch  Criteria=u2 > Threshold  SaturateOnIntegerOverflow=off  InputSameDT=off
  disarm motor : Subsystem
  mode_out : Outport
  battery_low_trigger : Outport  Port=2
  wires:
  mode_in/1 -> Switch/3
  Compare To Constant3/1 -> disarm motor/Enable
  voltage/1 -> Compare To Constant3/1
  disarm motor/1(battery_low_trigger) -> battery_low_trigger/1, Switch/2
  Switch/1 -> mode_out/1
  Constant/1 -> Switch/1

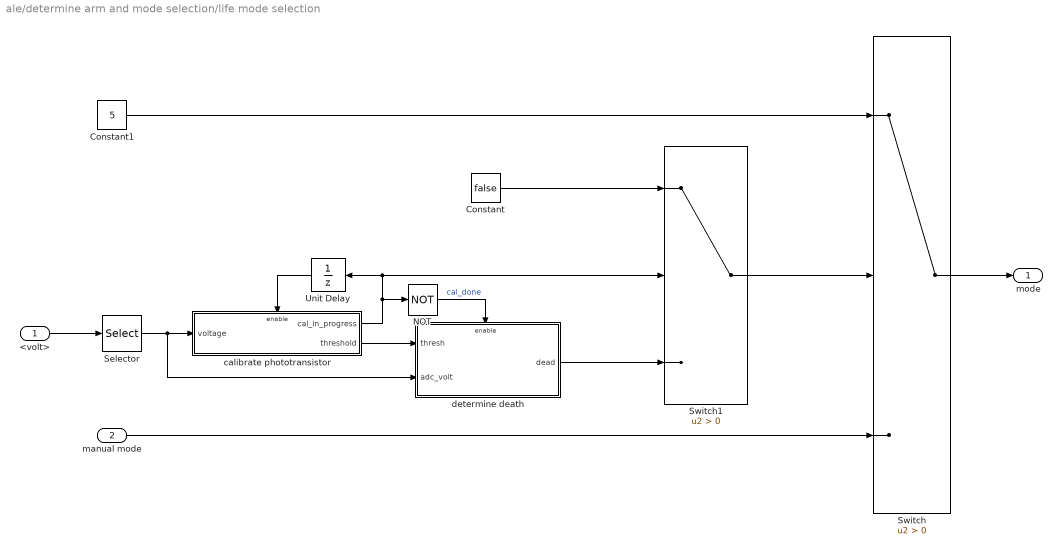
== system ale/determine arm and mode selection/life mode selection ==
  <volt> : Inport
  manual mode : Inport  Port=2
  Constant : Constant  Value=false
  Constant1 : Constant  Value=5  OutDataTypeStr=int8  SampleTime=framePeriod_s
  NOT : Logic  Operator=NOT  IconShape=distinctive  AllPortsSameDT=off  OutDataTypeStr=boolean
  Selector : Selector  InputPortWidth=2  IndexOptions=Index vector (dialog)  Indices=[1]  OutputSizes=1
  Switch : Switch  Criteria=u2 > Threshold  SaturateOnIntegerOverflow=off  InputSameDT=off
  Switch1 : Switch  Criteria=u2 > Threshold  SaturateOnIntegerOverflow=off  InputSameDT=off
  Unit Delay : UnitDelay  InitialCondition=true  SampleTime=-1  HasFrameUpgradeWarning=on
  calibrate phototransistor : Subsystem
  determine death : Subsystem
  mode : Outport
  wires:
  Constant1/1 -> Switch/1
  Switch/1 -> mode/1
  manual mode/1 -> Switch/3
  Selector/1 -> determine death/2(adc_volt), calibrate phototransistor/1(voltage)
  calibrate phototransistor/1(cal_in_progress) -> Switch1/2, Unit Delay/1, NOT/1
  calibrate phototransistor/2(threshold) -> determine death/1(thresh)
  determine death/1(dead) -> Switch1/3
  NOT/1 -> determine death/Enable  "cal_done"
  Switch1/1 -> Switch/2
  Constant/1 -> Switch1/1
  <volt>/1 -> Selector/1
  Unit Delay/1 -> calibrate phototransistor/Enable

== system ale/WAYPOINT CONTROLLER/WP_NAV/heading_controller ==
  navData : Inport
  cur_target_heading_rad : Inport  Port=2
  P_heading : Inport  Port=3
  Bus Selector4 : BusSelector  OutputSignals=heading_rad
  heading_controller : Subsystem
  yaw_rate_cmd_radps : Outport
  wires:
  navData/1 -> Bus Selector4/1
  cur_target_heading_rad/1 -> heading_controller/1(heading_cmd_rad)
  Bus Selector4/1 -> heading_controller/2(<heading_rad>)  "<heading_rad>"
  heading_controller/1(yaw_rate_cmd) -> yaw_rate_cmd_radps/1
  P_heading/1 -> heading_controller/3(p_heading)

== system ale/WAYPOINT CONTROLLER/WP_NAV/horizontal_error_calculation  ==
  target_pos_m : Inport
  cur_pos_m : Inport  Port=2
  Atan2 : Trigonometry  Operator=atan2
  Demux2 : Demux  Outputs=2
  MatrixMultiply : Product  Multiplication=Matrix(*)
  Selector : Selector  InputPortWidth=3  IndexOptions=Index vector (dialog)  Indices=[1 2]  OutputSizes=1
  Sqrt : Sqrt
  Subtract : Sum  Inputs=+-
  Transpose : Math  Operator=transpose
  dist_to_target_m : Outport
  bearing_to_tar_rad : Outport  Port=2
  wires:
  target_pos_m/1 -> Subtract/1
  cur_pos_m/1 -> Subtract/2
  Selector/1 -> Demux2/1, MatrixMultiply/2, Transpose/1
  Atan2/1 -> bearing_to_tar_rad/1
  Subtract/1 -> Selector/1
  Demux2/2 -> Atan2/1
  Transpose/1 -> MatrixMultiply/1
  MatrixMultiply/1 -> Sqrt/1
  Demux2/1 -> Atan2/2
  Sqrt/1 -> dist_to_target_m/1

== system ale/WAYPOINT CONTROLLER/determine target/calc_prev_target_pos ==
  prev_ind : Inport
  <flight_plan> : Inport  Port=2
  home_lat_rad : Inport  Port=3
  home_lon_rad : Inport  Port=4
  home_alt : Inport  Port=5
  Enable : EnablePort
  Bus Selector2 : BusSelector  OutputSignals=x,y,z
  Selector1 : Selector  IndexMode=Zero-based  InputPortWidth=100  IndexOptions=Index vector (port)  Indices=[1 3]  OutputSizes=1
  determine_prev_tar_pos : MATLAB Function  TreatAsAtomicUnit=on
  pref_target_pos : Outport
  wires:
  home_lon_rad/1 -> determine_prev_tar_pos/5(home_lon_rad)
  home_alt/1 -> determine_prev_tar_pos/6(home_alt)
  Bus Selector2/2 -> determine_prev_tar_pos/2(fp_y)  "<y>"
  home_lat_rad/1 -> determine_prev_tar_pos/4(home_lat_rad)
  prev_ind/1 -> Selector1/2
  <flight_plan>/1 -> Selector1/1
  determine_prev_tar_pos/1(prev_target_pos) -> pref_target_pos/1
  Bus Selector2/1 -> determine_prev_tar_pos/1(fp_x)  "<x>"
  Bus Selector2/3 -> determine_prev_tar_pos/3(fp_z)  "<z>"
  Selector1/1 -> Bus Selector2/1

== system ale/determine arm and mode selection/battery_failsafe/disarm motor ==
  Enable : EnablePort  StatesWhenEnabling=reset
  Compare To Constant2 : simulink/Logic and Bit Operations/Compare To Constant  relop=>  const=15  OutDataTypeStr=boolean
  Constant : Constant  Value=framePeriod_s
  Sum : Sum  Inputs=|++
  Unit Delay : UnitDelay  SampleTime=-1  HasFrameUpgradeWarning=on
  battery_low_trigger : Outport
  wires:
  Compare To Constant2/1 -> battery_low_trigger/1
  Sum/1 -> Compare To Constant2/1, Unit Delay/1
  Unit Delay/1 -> Sum/2
  Constant/1 -> Sum/1

== system ale/determine arm and mode selection/life mode selection/calibrate phototransistor ==
  voltage : Inport
  Enable : EnablePort
  Compare To Constant : simulink/Logic and Bit Operations/Compare To Constant  relop=<  const=Aircraft.Sensors.phototransistor.cal_count  OutDataTypeStr=boolean
  Multiply : Gain  Gain=1 + Aircraft.Control.death_buffer
  average voltage : Subsystem
  counter : Subsystem
  cal_in_progress : Outport
  threshold : Outport  Port=2
  wires:
  Compare To Constant/1 -> cal_in_progress/1
  Multiply/1 -> threshold/1
  voltage/1 -> average voltage/1(In1)
  average voltage/1(Out1) -> Multiply/1
  counter/1(iterations) -> Compare To Constant/1

== system ale/determine arm and mode selection/life mode selection/determine death ==
  thresh : Inport
  adc_volt : Inport  Port=2
  Enable : EnablePort
  MATLAB Function : MATLAB Function  TreatAsAtomicUnit=on
  dead : Outport
  wires:
  MATLAB Function/1(dead) -> dead/1
  thresh/1 -> MATLAB Function/1(thresh)
  adc_volt/1 -> MATLAB Function/2(adc_volt)
